simulink model "Task21"  (R2025a)
settings: Solver=VariableStepAuto  StartTime=0.0  StopTime=10.0  RelTol=1e-3
settings Model: Creator=LOQ  LastModifiedBy=LOQ

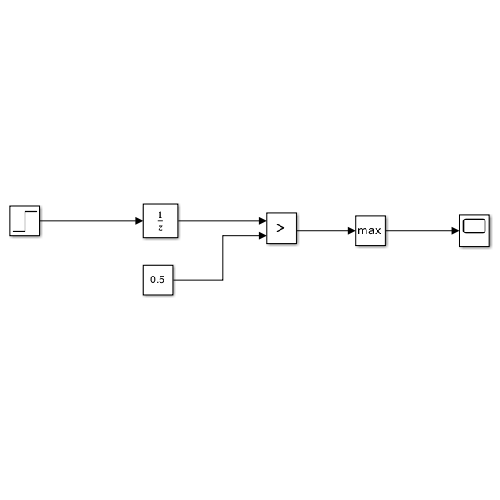
[thumbnail: Simulink's stored preview of the top-level diagram]
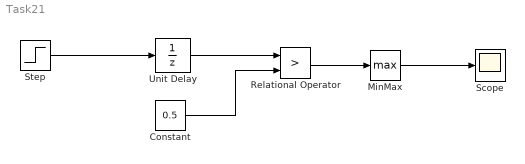
== system Task21 ==
  Constant : Constant  Value=0.5
  MinMax : MinMax  Function=max
  Relational Operator : RelationalOperator  Operator=>  OutDataTypeStr=boolean  RndMeth=Simplest  InputSameDT=off
  Scope : Scope
      settings: ActiveDisplayYMinimum=-0.12499999999999997  ActiveDisplayYMaximum=1.125
  Step : Step  Time=2  After=10  SampleTime=0
  Unit Delay : UnitDelay  SampleTime=-1  HasFrameUpgradeWarning=on
  wires:
  Step/1 -> Unit Delay/1
  Unit Delay/1 -> Relational Operator/1
  Constant/1 -> Relational Operator/2
  Relational Operator/1 -> MinMax/1
  MinMax/1 -> Scope/1
